simulink model "TRAMI_DTTH_PNT"  (R2018b)
settings: Solver=ode8  StartTime=0  StopTime=end_time  FixedStep=0.001  RelTol=1e-3
PreLoadFcn:
  | TRAMI_DTTH_PNT_PreLoad;
settings Model: Creator=nishimura  LastModifiedBy=E00026
settings DataIOCC: LimitDataPoints=on  SaveFormat=Array  SaveOutput=off  InspectSignalLogs=on  SaveTime=off
settings OptimizationCC: BlockReduction=off  BooleanDataType=off  LifeSpan=inf
settings DebuggingCC: SaveWithParameterizedLinksMsg=none  UnderspecifiedInitializationDetection=Classic  MergeDetectMultiDrivingBlocksExec=none  SignalResolutionControl=TryResolveAllWithWarning  ParameterPrecisionLossMsg=none  StrictBusMsg=ErrorOnBusTreatedAsVector  SFUnexpectedBacktrackingDiag=warning  SFNoUnconditionalDefaultTransitionDiag=warning  SFExecutionAtInitializationDiag=none
settings HardwareCC: ProdBitPerPointer=32  ProdBitPerSizeT=32  ProdBitPerPtrDiffT=32  ProdLargestAtomicFloat=None  ProdIntDivRoundTo=Undefined  ProdEndianess=Unspecified  ProdWordSize=32  ProdHWDeviceType=32-bit Generic  TargetUnknown=on
settings ModelReferenceCC: PropagateSignalLabelsOutOfModel=off
settings SFSimCC: SimUseLocalCustomCode=off
settings RTWCC: RTWUseLocalCustomCode=off
settings CodeAppCC: StateflowObjectComments=on
settings GRTTargetCC: TargetLangStandard=C89/C90 (ANSI)  GeneratePreprocessorConditionals=Disable all
settings ConfigComp: CovMetricSettings=dw  CovHtmlReporting=on  CovSaveCumulativeToWorkspaceVar=on  CovSaveSingleToWorkspaceVar=on  CovExternalEMLEnable=off  CovSFcnEnable=off

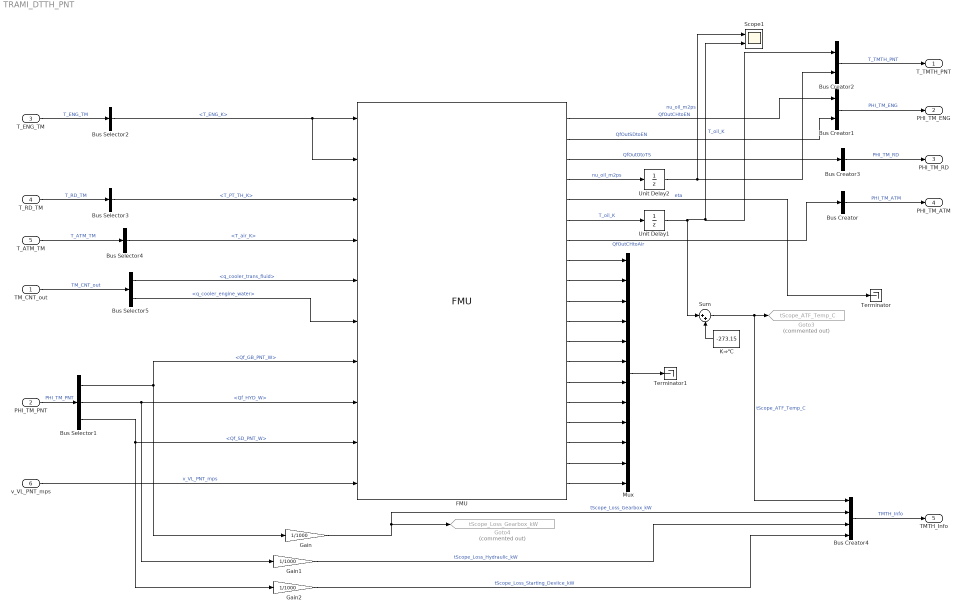
== system TRAMI_DTTH_PNT ==
  TM_CNT_out : Inport  OutDataTypeStr=Bus: TM_CNT_out  SampleTime=[0.001,0]
      settings: AttributesFormatString=|
      | <SampleTime = %<SampleTime>>
      | <%<OutDataTypeStr>>
  PHI_TM_PNT : Inport  Port=2  OutDataTypeStr=Bus: PHI_TM_PNT  SampleTime=[0.001,0]
      settings: AttributesFormatString=|
      | <SampleTime = %<SampleTime>>
      | <%<OutDataTypeStr>>
  T_ENG_TM : Inport  Port=3  OutDataTypeStr=Bus: T_ENG_TM  SampleTime=0
      settings: AttributesFormatString=|
      | <SampleTime = %<SampleTime>>
      | <%<OutDataTypeStr>>
  T_RD_TM : Inport  Port=4  OutDataTypeStr=Bus: T_RD_TM  SampleTime=0
      settings: AttributesFormatString=|
      | <SampleTime = %<SampleTime>>
      | <%<OutDataTypeStr>>
  T_ATM_TM : Inport  Port=5  OutDataTypeStr=Bus: T_ATM_TM  SampleTime=0
      settings: AttributesFormatString=|
      | <SampleTime = %<SampleTime>>
      | <%<OutDataTypeStr>>
  v_VL_PNT_mps : Inport  Port=6  OutDataTypeStr=double  PortDimensions=1  SampleTime=0
      settings: AttributesFormatString=<SampleTime = %<SampleTime>>
  Bus Creator : BusCreator  Inputs=1
  Bus Creator1 : BusCreator  Inputs=2
  Bus Creator2 : BusCreator  Inputs=2
  Bus Creator3 : BusCreator  Inputs=1
  Bus Creator4 : BusCreator  Inputs=4
  Bus Selector1 : BusSelector  OutputSignals=Qf_GB_PNT_W,Qf_HYD_W,Qf_SD_PNT_W
  Bus Selector2 : BusSelector  OutputSignals=T_ENG_K
  Bus Selector3 : BusSelector  OutputSignals=T_PT_TH_K
  Bus Selector4 : BusSelector  OutputSignals=T_air_K
  Bus Selector5 : BusSelector  OutputSignals=q_cooler_trans_fluid,q_cooler_engine_water
  FMU : FMU  FMUName=ThermalModelAll_CS.fmu  FMUDebugLogging=on  FMUMode=CoSimulation  c1=5000  T0=300  R1=100  T1=300  R2=0.10  R3=100  R4=100  R5=0.006  table1_1_1__1_1_=0.  table1_1_2__1_2_=0.022  table1_2_1__2_1_=10.  table1_2_2__2_2_=0.021  table1_3_1__3_1_=20.  table1_3_2__3_2_=0.021  table1_4_1__4_1_=30.  table1_4_2__4_2_=0.020  table1_5_1__5_1_=40.  table1_5_2__5_2_=0.019  table1_6_1__6_1_=50.  table1_6_2__6_2_=0.018  table1_7_1__7_1_=60.  table1_7_2__7_2_=0.017  table1_8_1__8_1_=70.  table1_8_2__8_2_=0.016  table1_9_1__9_1_=80.  table1_9_2__9_2_=0.015  table1_10_1__10_1_=90.  table1_10_2__10_2_=0.014  table1_11_1__11_1_=100.  table1_11_2__11_2_=0.013  table1_12_1__12_1_=110.  table1_12_2__12_2_=0.012  table1_13_1__13_1_=120.  table1_13_2__13_2_=0.012  table1_14_1__14_1_=130.  table1_14_2__14_2_=0.011  table1_15_1__15_1_=140.  table1_15_2__15_2_=0.011  table1_16_1__16_1_=150.  table1_16_2__16_2_=0.010  table1_17_1__17_1_=160.  table1_17_2__17_2_=0.010  c3=15000  T2=300  fileName1=./DATA/thResistanceOilColler1.txt  tableName1=thResistanceOilColler1  T3=300  c4=10000  R6=0.0007  R7=0.05  Nutable1_1_1__1_1_=-30.  Nutable1_1_2__1_2_=70  Nutable1_2_1__2_1_=0.  Nutable1_2_2__2_2_=70  Nutable1_3_1__3_1_=20.  Nutable1_3_2__3_2_=70  Nutable1_4_1__4_1_=40.  Nutable1_4_2__4_2_=40  Nutable1_5_1__5_1_=60.  Nutable1_5_2__5_2_=23  Nutable1_6_1__6_1_=80.  Nutable1_6_2__6_2_=13  Nutable1_7_1__7_1_=100.  Nutable1_7_2__7_2_=7.5  Nutable1_8_1__8_1_=120.  Nutable1_8_2__8_2_=7.5  EtaTable1_1_1__1_1_=-30.  EtaTable1_1_2__1_2_=70  EtaTable1_2_1__2_1_=0.  EtaTable1_2_2__2_2_=70  EtaTable1_3_1__3_1_=20.  EtaTable1_3_2__3_2_=70  EtaTable1_4_1__4_1_=40.  EtaTable1_4_2__4_2_=40  EtaTable1_5_1__5_1_=60.  EtaTable1_5_2__5_2_=23  EtaTable1_6_1__6_1_=80.  EtaTable1_6_2__6_2_=13  EtaTable1_7_1__7_1_=100.  EtaTable1_7_2__7_2_=7.5  EtaTable1_8_1__8_1_=120.  EtaTable1_8_2__8_2_=7.5  kDammy=1.  c2=30000  settings_dtMin=1e-08  settings_dtMax=0.01  settings_absTol=1e-05  settings_relTol=1e-05  settings_iMode=int32(1)  settings_maxOrder=int32(5)  mask(ThermalModelAll [Co-Simulation, v2.0]){}
      mask Display:
      | disp('ThermalModelAll');
      | port_label('output',1,'QfOutCHtoEN');
      | port_label('output',2,'QfOutSDtoEN');
      | port_label('output',3,'QfOutOCtoTS');
      | port_label('output',4,'nuOil');
      | port_label('output',5,'etaOil');
      | port_label('output',6,'ToutOil');
      | port_label('output',7,'QfOutCHtoAir');
      | port_label('output',8,'ToutOiltoOC');
      | port_label('output',9,'QfOutOCtoOil');
      | port_label('output',10,'ToutSDtoOil');
      | port_label('output',11,'QfOutOiltoSD');
      | port_label('output',12,'ToutSDtoCH');
      | port_label('output',13,'QfOutCHtoSD');
      | port_label('output',14,'ToutOiltoCH');
      | port_label('output',15,'QfoutCHtoOil');
      | port_label('output',16,'QfOiltoGear');
      | port_label('output',17,'ToutGeartoOil');
      | port_label('output',18,'ToutGeartoCH');
      | port_label('output',19,'QfOutCHtoGear');
      | port_label('input',1,'TinENtoCH');
      | port_label('input',2,'TinENtoSD');
      | port_label('input',3,'TinTStoOC');
      | port_label('input',4,'TinAirtoCH');
      | port_label('input',5,'VIdot1OilCooler');
      | port_label('input',6,'VIdot2OilCooler');
      | port_label('input',7,'QfGear');
      | port_label('input',8,'QfOil');
      | port_label('input',9,'QfStartDevice');
      | port_label('input',10,'vCaseHousing');
  Gain : Gain  Gain=1/1000
  Gain1 : Gain  Gain=1/1000
  Gain2 : Gain  Gain=1/1000
  Goto3 : Goto  Commented=on  GotoTag=tScope_ATF_Temp_C  TagVisibility=global
  Goto4 : Goto  Commented=on  GotoTag=tScope_Loss_Gearbox_kW  TagVisibility=global
  K⇒℃ : Constant  Value=-273.15
  Mux : Mux  Inputs=12
  Scope1 : Scope  NumInputPorts=2
  Sum : Sum  Inputs=|++
  Terminator : Terminator
  Terminator1 : Terminator
  Unit Delay1 : UnitDelay  InitialCondition=8e-5  SampleTime=-1
  Unit Delay2 : UnitDelay  InitialCondition=8e-5  SampleTime=-1
  T_TMTH_PNT : Outport  OutDataTypeStr=Bus: T_TMTH_PNT  SampleTime=[0.001,0]
      settings: AttributesFormatString=<%<OutDataTypeStr>>
  PHI_TM_ENG : Outport  Port=2  OutDataTypeStr=Bus: PHI_TM_ENG  SampleTime=[0.001,0]
      settings: AttributesFormatString=<%<OutDataTypeStr>>
  PHI_TM_RD : Outport  Port=3  OutDataTypeStr=Bus: PHI_TM_RD  SampleTime=[0.001,0]
      settings: AttributesFormatString=<%<OutDataTypeStr>>
  PHI_TM_ATM : Outport  Port=4  OutDataTypeStr=Bus: PHI_TM_ATM  SampleTime=[0.001,0]
      settings: AttributesFormatString=<%<OutDataTypeStr>>
  TMTH_Info : Outport  Port=5  OutDataTypeStr=Bus: TMTH_Info  SampleTime=[0.001,0]
      settings: AttributesFormatString=<%<OutDataTypeStr>>
  wires:
  Bus Selector1/1 -> FMU/7, Gain/1  "<Qf_GB_PNT_W>"
  Unit Delay2/1 -> Bus Creator2/2, Scope1/1  "nu_oil_m2ps"
  Bus Creator4/1 -> TMTH_Info/1  "TMTH_Info"
  Unit Delay1/1 -> Sum/1, Scope1/2, Bus Creator2/1  "T_oil_K"
  FMU/18 -> Mux/11
  Sum/1 -> Goto3/1, Bus Creator4/1  "tScope_ATF_Temp_C"
  FMU/14 -> Mux/7
  T_ENG_TM/1 -> Bus Selector2/1  "T_ENG_TM"
  Gain/1 -> Goto4/1, Bus Creator4/2  "tScope_Loss_Gearbox_kW"
  Mux/1 -> Terminator1/1
  FMU/7 -> Bus Creator/1  "QfOutCHtoAir"
  Bus Creator1/1 -> PHI_TM_ENG/1  "PHI_TM_ENG"
  Bus Selector1/2 -> Gain1/1, FMU/8  "<Qf_HYD_W>"
  v_VL_PNT_mps/1 -> FMU/10  "v_VL_PNT_mps"
  FMU/1 -> Bus Creator1/1  "QfOutCHtoEN"
  TM_CNT_out/1 -> Bus Selector5/1  "TM_CNT_out"
  FMU/6 -> Unit Delay1/1  "T_oil_K"
  Bus Selector1/3 -> FMU/9, Gain2/1  "<Qf_SD_PNT_W>"
  T_RD_TM/1 -> Bus Selector3/1  "T_RD_TM"
  Bus Selector5/1 -> FMU/5  "<q_cooler_trans_fluid>"
  Bus Creator/1 -> PHI_TM_ATM/1  "PHI_TM_ATM"
  FMU/9 -> Mux/2
  FMU/11 -> Mux/4
  PHI_TM_PNT/1 -> Bus Selector1/1  "PHI_TM_PNT"
  Bus Selector2/1 -> FMU/1, FMU/2  "<T_ENG_K>"
  K⇒℃/1 -> Sum/2
  FMU/16 -> Mux/9
  FMU/15 -> Mux/8
  FMU/10 -> Mux/3
  FMU/2 -> Bus Creator1/2  "QfOutSDtoEN"
  FMU/8 -> Mux/1
  FMU/13 -> Mux/6
  Bus Selector5/2 -> FMU/6  "<q_cooler_engine_water>"
  FMU/19 -> Mux/12
  FMU/17 -> Mux/10
  FMU/12 -> Mux/5
  T_ATM_TM/1 -> Bus Selector4/1  "T_ATM_TM"
  FMU/5 -> Terminator/1  "eta"
  Bus Selector4/1 -> FMU/4  "<T_air_K>"
  FMU/3 -> Bus Creator3/1  "QfOutOtoTS"
  FMU/4 -> Unit Delay2/1  "nu_oil_m2ps"
  Bus Creator2/1 -> T_TMTH_PNT/1  "T_TMTH_PNT"
  Gain1/1 -> Bus Creator4/3  "tScope_Loss_Hydraulic_kW"
  Bus Selector3/1 -> FMU/3  "<T_PT_TH_K>"
  Gain2/1 -> Bus Creator4/4  "tScope_Loss_Starting_Deviice_kW"
  Bus Creator3/1 -> PHI_TM_RD/1  "PHI_TM_RD"
